simulink model "A227"  (R2018b)
settings: Solver=VariableStepAuto  StartTime=0.0  StopTime=10.0  RelTol=1e-3
libraries: arduinolib x1, dspstat3 x1, simulink x1
settings Model: Creator=bill  LastModifiedBy=bill

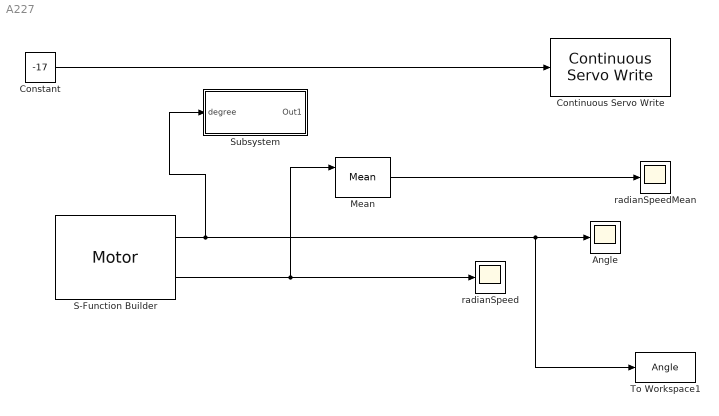
== system A227 ==
  Angle : Scope
  Constant : Constant  Value=-17
  Continuous Servo Write : arduinolib/Continuous Servo Write  pinNumber=7  ServoIndex=0  blockPlatform=ARDUINO
      settings: SourceProductName=Simulink Support Package for Arduino Hardware  SourceProductBaseCode=ARDUINO
  Mean : dspstat3/Mean  run=on  InputProcessing=Columns as channels (frame based)  reset_popup=Rising edge  directionMode=Each column  dimension=1  roiEnable=off  roiType=Rectangles  roiPortion=Entire ROI  roiOutput=Individual statistics for each ROI  roiFlag=off  roundingMode=Floor  overflowMode=off  outputDataTypeStr=Inherit: Same as accumulator  outputMin=[]  outputMax=[]  outputLastDataTypeStr=Inherit: Same as accumulator
  S-Function Builder : S-Function  InitFcn=try, set_param(gcb,'FunctionName','Motor'), end  FunctionName=Motor  SFunctionModules=Motor_wrapper  SFunctionDeploymentMode=off  EnableBusSupport=off  mask(S-Function Builder){}
      mask help: Simulink:masks:SFunctionBuilder_MD
      mask init:
      | val = [[.9  0.75 0.75 1 1 .9 .9 1]',[1 1 0.75 0.75 .9 .9 1 .9]'];try , sys = get_param(gcb,'SfunBuilderFcnName');if isempty(sys), sys = get_param(gcb,'FunctionName'); end,catch, sys = get_param(gcb,'FunctionName'); end
      settings: CopyFcn=set_param(gcbh,'LinkStatus','none')  PreSaveFcn=try, set_param(gcb,'FunctionName','Motor'), end  OpenFcn=sfunctionwizard(gcbh)
      mask Display: plot(val(:,1),val(:,2)),disp(sys), port_label('output',1,'posRad'), port_label('output',2,'deriv')
  Subsystem : Subsystem
  To Workspace1 : ToWorkspace  VariableName=Angle  SampleTime=-1
  radianSpeed : Scope
  radianSpeedMean : Scope
  wires:
  Mean/1 -> radianSpeedMean/1
  S-Function Builder/1 -> Subsystem/1(degree), To Workspace1/1, Angle/1
  S-Function Builder/2 -> Mean/1, radianSpeed/1
  Constant/1 -> Continuous Servo Write/1

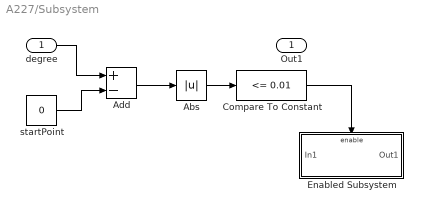
== system A227/Subsystem ==
  degree : Inport
  Abs : Abs
  Add : Sum  Inputs=+-
  Compare To Constant : simulink/Logic and Bit Operations/Compare To Constant  relop=<=  const=0.01  OutDataTypeStr=boolean
  Enabled Subsystem : Subsystem  TreatAsAtomicUnit=on
  startPoint : Constant  Value=0
  Out1 : Outport
  wires:
  degree/1 -> Add/1
  startPoint/1 -> Add/2
  Add/1 -> Abs/1
  Abs/1 -> Compare To Constant/1
  Compare To Constant/1 -> Enabled Subsystem/Enable

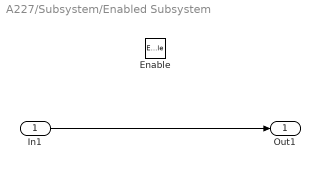
== system A227/Subsystem/Enabled Subsystem ==
  In1 : Inport
  Enable : EnablePort
  Out1 : Outport
  wires:
  In1/1 -> Out1/1
